simulink library "AEBSFunctionLib"  (R2021a)
settings: Solver=VariableStepAuto  StartTime=0.0  StopTime=10.0  RelTol=1e-3
settings Model: Creator=Acer  LastModifiedBy=jiapengfei
settings SolverCC: AlgebraicLoopSolver=TrustRegion
settings DataIOCC: ReturnWorkspaceOutputs=off
settings DebuggingCC: SFMachineParentedDataDiag=warning  ArithmeticOperatorsInVariantConditions=warning
settings SFSimCC: SimUseLocalCustomCode=off  CustomCodeUndefinedFunction=UseInterfaceOnly
settings RTWCC: RTWUseLocalCustomCode=off
settings CodeAppCC: StateflowObjectComments=on

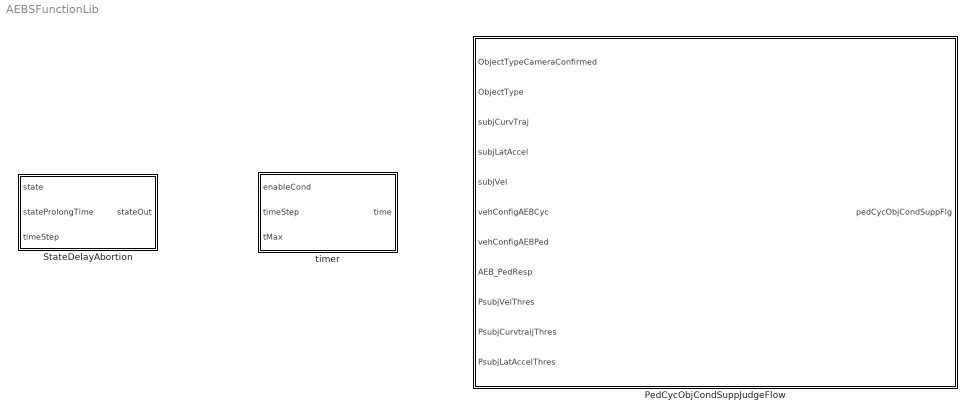
== system AEBSFunctionLib ==
  PedCycObjCondSuppJudgeFlow : Subsystem  TreatAsAtomicUnit=on
  StateDelayAbortion : Subsystem  TreatAsAtomicUnit=on
  timer : Subsystem  TreatAsAtomicUnit=on

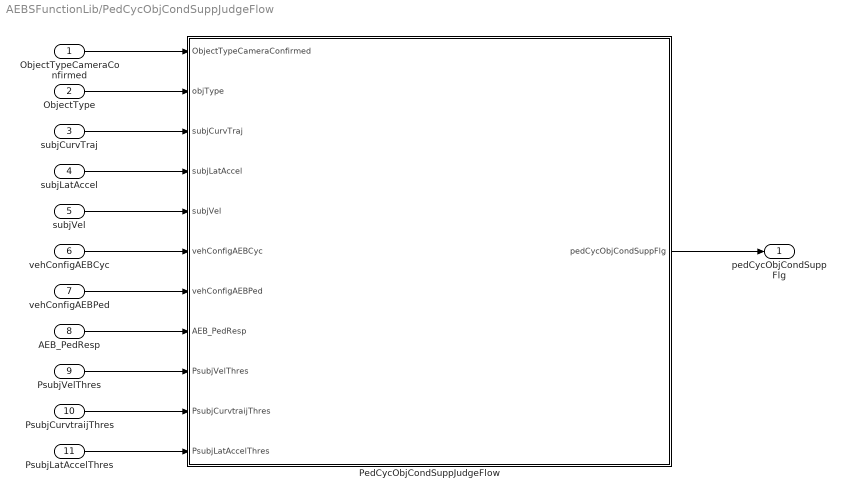
== system AEBSFunctionLib/PedCycObjCondSuppJudgeFlow ==
  ObjectTypeCameraConfirmed : Inport
  ObjectType : Inport  Port=2
  subjCurvTraj : Inport  Port=3
  subjLatAccel : Inport  Port=4
  subjVel : Inport  Port=5
  vehConfigAEBCyc : Inport  Port=6
  vehConfigAEBPed : Inport  Port=7
  AEB_PedResp : Inport  Port=8
  PsubjVelThres : Inport  Port=9
  PsubjCurvtraijThres : Inport  Port=10
  PsubjLatAccelThres : Inport  Port=11
  PedCycObjCondSuppJudgeFlow : Stateflow chart  TreatAsAtomicUnit=on
  pedCycObjCondSuppFlg : Outport
  wires:
  PsubjLatAccelThres/1 -> PedCycObjCondSuppJudgeFlow/11(PsubjLatAccelThres)
  PsubjCurvtraijThres/1 -> PedCycObjCondSuppJudgeFlow/10(PsubjCurvtraijThres)
  PedCycObjCondSuppJudgeFlow/1(pedCycObjCondSuppFlg) -> pedCycObjCondSuppFlg/1
  vehConfigAEBCyc/1 -> PedCycObjCondSuppJudgeFlow/6(vehConfigAEBCyc)
  subjLatAccel/1 -> PedCycObjCondSuppJudgeFlow/4(subjLatAccel)
  subjVel/1 -> PedCycObjCondSuppJudgeFlow/5(subjVel)
  ObjectType/1 -> PedCycObjCondSuppJudgeFlow/2(objType)
  AEB_PedResp/1 -> PedCycObjCondSuppJudgeFlow/8(AEB_PedResp)
  subjCurvTraj/1 -> PedCycObjCondSuppJudgeFlow/3(subjCurvTraj)
  vehConfigAEBPed/1 -> PedCycObjCondSuppJudgeFlow/7(vehConfigAEBPed)
  PsubjVelThres/1 -> PedCycObjCondSuppJudgeFlow/9(PsubjVelThres)
  ObjectTypeCameraConfirmed/1 -> PedCycObjCondSuppJudgeFlow/1(ObjectTypeCameraConfirmed)

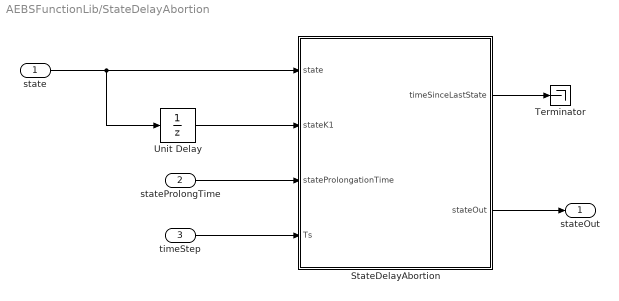
== system AEBSFunctionLib/StateDelayAbortion ==
  state : Inport
  stateProlongTime : Inport  Port=2
  timeStep : Inport  Port=3
  StateDelayAbortion : Stateflow chart  TreatAsAtomicUnit=on
  Terminator : Terminator
  Unit Delay : UnitDelay  SampleTime=-1  HasFrameUpgradeWarning=on
  stateOut : Outport
  wires:
  state/1 -> Unit Delay/1, StateDelayAbortion/1(state)
  Unit Delay/1 -> StateDelayAbortion/2(stateK1)
  stateProlongTime/1 -> StateDelayAbortion/3(stateProlongationTime)
  timeStep/1 -> StateDelayAbortion/4(Ts)
  StateDelayAbortion/1(timeSinceLastState) -> Terminator/1
  StateDelayAbortion/2(stateOut) -> stateOut/1

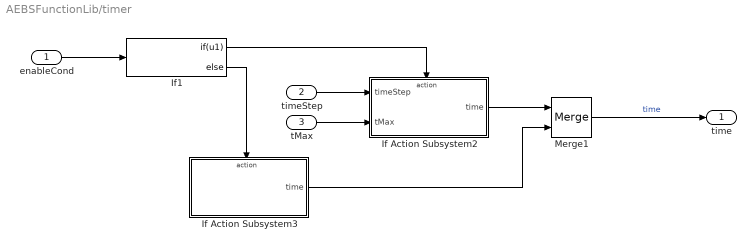
== system AEBSFunctionLib/timer ==
  enableCond : Inport
  timeStep : Inport  Port=2
  tMax : Inport  Port=3
  If Action Subsystem2 : Subsystem  TreatAsAtomicUnit=on
  If Action Subsystem3 : Subsystem  TreatAsAtomicUnit=on
  If1 : If  IfExpression=u1
  Merge1 : Merge
  time : Outport
  wires:
  If1/1 -> If Action Subsystem2/Action
  If Action Subsystem2/1(time) -> Merge1/1
  If1/2 -> If Action Subsystem3/Action
  If Action Subsystem3/1(time) -> Merge1/2
  enableCond/1 -> If1/1
  timeStep/1 -> If Action Subsystem2/1(timeStep)
  Merge1/1 -> time/1  "time"
  tMax/1 -> If Action Subsystem2/2(tMax)

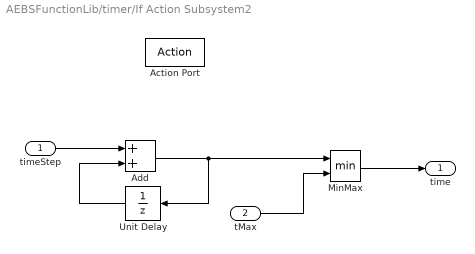
== system AEBSFunctionLib/timer/If Action Subsystem2 ==
  timeStep : Inport
  tMax : Inport  Port=2
  Action Port : ActionPort  InitializeStates=reset
  Add : Sum
  MinMax : MinMax  Inputs=2
  Unit Delay : UnitDelay  SampleTime=-1  HasFrameUpgradeWarning=on
      settings: AttributesFormatString=InitialCondition:%<InitialCondition>
  time : Outport
  wires:
  Add/1 -> Unit Delay/1, MinMax/1
  tMax/1 -> MinMax/2
  MinMax/1 -> time/1
  timeStep/1 -> Add/1
  Unit Delay/1 -> Add/2

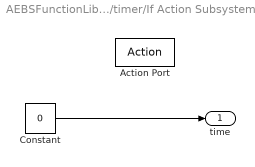
== system AEBSFunctionLib/timer/If Action Subsystem3 ==
  Action Port : ActionPort
  Constant : Constant  Value=0
  time : Outport
  wires:
  Constant/1 -> time/1

== stateflow chart AEBSFunctionLib/PedCycObjCondSuppJudgeFlow/PedCycObjCondSuppJudgeFlow ==
  (default) -> (junction 2)
  (junction 2) -> (junction 3) [order 1] : [objType == ObjectTypeCopy.PEDESTRIAN ||...
      | objType == ObjectTypeCopy.BICYCLE]
  (junction 2) -> (junction 7) [order 2] : {
      | 	pedCycObjCondSuppFlg = false;
      | }
  (junction 3) -> (junction 5)
  (junction 5) -> (junction 9) [order 1] : [abs(subjCurvTraj) > PsubjCurvtraijThres ||...
      | abs(subjLatAccel) > PsubjLatAccelThres]
  (junction 5) -> (junction 13) [order 2] : {
      | 	subjDrvCondSuppFlg = false;
      | }
  (junction 9) -> (junction 11) : {
      | 	subjDrvCondSuppFlg = true;
      | }
  (junction 11) -> (junction 13)
  (junction 13) -> (junction 16)
  (junction 16) -> (junction 18) [order 1] : [subjVel > PsubjVelThres ||...
      | ObjectTypeCameraConfirmed == false ||...
      | subjDrvCondSuppFlg == true || ...
      | AEB_PedResp == CNSwtOFF ||...
      | vehConfigAEBPed == false ||...
      | vehConfigAEBCyc == false]
  (junction 16) -> (junction 22) [order 2] : {
      | 	pedCycObjCondSuppFlg = false;
      | }
  (junction 18) -> (junction 20) : {
      | 	pedCycObjCondSuppFlg = true;
      | }
  (junction 22) -> (junction 7)
  (junction 20) -> (junction 22)
  (junction 7) -> (junction 26)
  data: ObjectTypeCameraConfirmed input; objType input Enum: ObjectTypeCopy; subjCurvTraj input; subjLatAccel input; subjVel input; vehConfigAEBCyc input; vehConfigAEBPed input; AEB_PedResp input; pedCycObjCondSuppFlg output; CNSwtOFF parameter; PsubjVelThres input; PsubjCurvtraijThres input; PsubjLatAccelThres input; subjDrvCondSuppFlg local boolean

== stateflow chart AEBSFunctionLib/StateDelayAbortion/StateDelayAbortion ==
  state NormalState
    en:
    stateOut = state;
    CNTimeCounterMAX = 256;
    du:
    stateOut = state;
  state CounterState
    en:
    timeSinceLastState = 0;
    du:
    timeSinceLastState +=  Ts;
    CounterStateFunc();
  state CounterStateFunc [function]
    (default) -> (junction 70)
    (junction 70) -> (junction 62) [order 1] : [timeSinceLastState > CNTimeCounterMAX]
    (junction 70) -> (junction 69) [order 2] : %do nothing
    (junction 62) -> (junction 61) : {
        | 	timeSinceLastState = CNTimeCounterMAX;
        | }
    (junction 61) -> (junction 69)
    (junction 69) -> (junction 68)
    (junction 68) -> (junction 60) [order 1] : [timeSinceLastState < stateProlongationTime]
    (junction 68) -> (junction 66) [order 2] : {
        | 	stateOut = false;
        | }
    (junction 60) -> (junction 67) : {
        | 	stateOut = true;
        | }
    (junction 67) -> (junction 66)
    (junction 66) -> (junction 56)
  (default) -> NormalState
  NormalState -> CounterState : [stateK1 == true &&...
      | state == false]
  CounterState -> NormalState : [timeSinceLastState > stateProlongationTime]
  data: state input; stateK1 input; stateProlongationTime input; timeSinceLastState output double; stateOut output boolean; Ts input; CNTimeCounterMAX local double
